simulink model "Progetto_PREDISTORTER_Aggiornato_15_021"  (R2024b)
settings: Solver=VariableStepAuto  StartTime=0.0  StopTime=10  RelTol=1e-3
libraries: commrflib2 x5, commfilt2 x1
settings Model: Creator=babu9  LastModifiedBy=Giorgio
settings SolverCC: AlgebraicLoopSolver=TrustRegion
settings RTWCC: GPUComputeCapability=3.5  DLArmComputeVersion=19.05

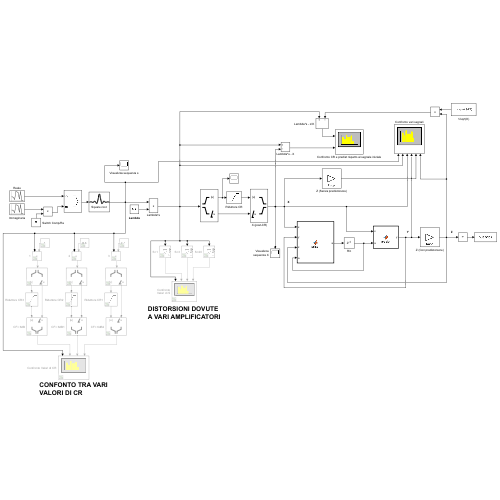
[thumbnail: Simulink's stored preview of the top-level diagram]
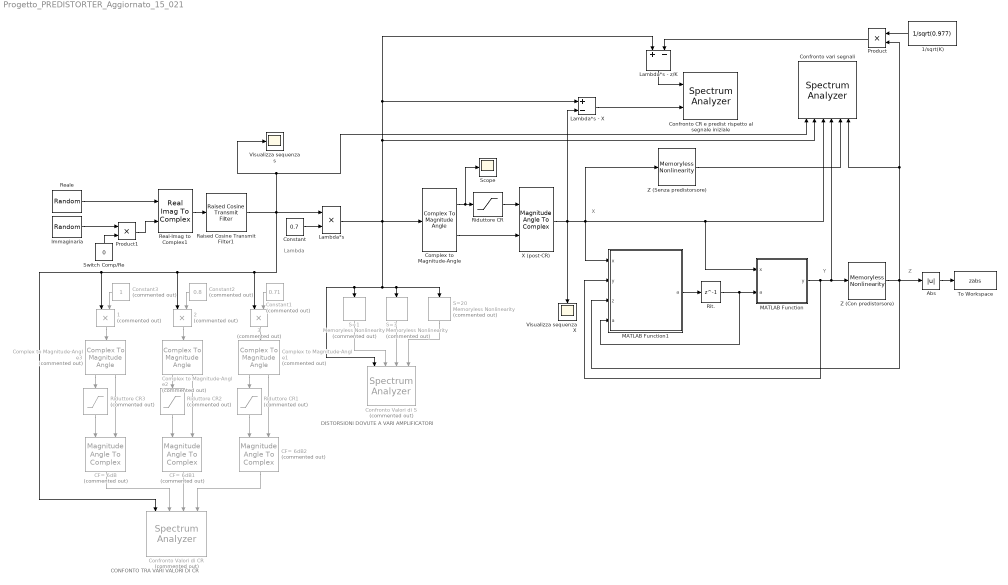
== system Progetto_PREDISTORTER_Aggiornato_15_021 ==
  note: DISTORSIONI DOVUTE
      | A VARI AMPLIFICATORI
  note: Lambda
  note: CONFONTO TRA VARI
      | VALORI DI CR
  note: Y
  note: Z
  note: X
  " X (post-CR)" : MagnitudeAngleToComplex
  1 : Product  Commented=on
  1/sqrt(K) : Constant  Value=1/sqrt(0.977)
  2 : Product  Commented=on
  3 : Product  Commented=on
  Abs : Abs  SaturateOnIntegerOverflow=off
  CF= 6dB : MagnitudeAngleToComplex  Commented=on
  CF= 6dB1 : MagnitudeAngleToComplex  Commented=on
  CF= 6dB2 : MagnitudeAngleToComplex  Commented=on
  Complex to Magnitude-Angle : ComplexToMagnitudeAngle
  Complex to Magnitude-Angle1 : ComplexToMagnitudeAngle  Commented=on
  Complex to Magnitude-Angle2 : ComplexToMagnitudeAngle  Commented=on
  Complex to Magnitude-Angle3 : ComplexToMagnitudeAngle  Commented=on
  Confronto Valori di S : SpectrumAnalyzer  Commented=on  NumInputPorts=4  AveragingMethod=Exponential  ShowLegend=on  ChannelNames="[\"\"]"  AllowFFTLengthLessThanSamplesPerUpdate=on  DefaultConfigurationName=spbscopes.SpectrumAnalyzerBlockCfg
  Confronto CR e predist rispetto al segnale iniziale : SpectrumAnalyzer  NumInputPorts=2  WindowPosition=[206.000000,154.000000,1536.000000,800.000000,]  ScopeFrameLocation=window  Span=8000  StartFrequency=-4000  StopFrequency=4000  AveragingMethod=Exponential  YLimits=[-58.97153624,-16.65787258]  ShowLegend=on  ChannelNames="[\"\"]"  AllowFFTLengthLessThanSamplesPerUpdate=on  DefaultConfigurationName=spbscopes.SpectrumAnalyzerBlockCfg
      settings: OpenAtSimulationStart=off
  Confronto Valori di CR : SpectrumAnalyzer  Commented=on  NumInputPorts=4  AveragingMethod=Exponential  ShowLegend=on  ChannelNames="[\"\"]"  AllowFFTLengthLessThanSamplesPerUpdate=on  DefaultConfigurationName=spbscopes.SpectrumAnalyzerBlockCfg
      settings: OpenAtSimulationStart=off
  Confronto vari segnali : SpectrumAnalyzer  NumInputPorts=6  WindowPosition=[257.000000,133.000000,1532.000000,791.000000,]  ScopeFrameLocation=window  SpectrumType=Power density  Span=80000  StartFrequency=-40000  StopFrequency=40000  AveragingMethod=Exponential  YLimits=[-146.14127615,3.33371478]  ShowLegend=on  ChannelNames="[\"s\", \"Lambda*s\", \"X post-CR\", \"Y (Uscita predistorsore)\", \"Z - Senza predistorsore\", \"Z - Con predistorsore\"]"  MeasurementChannel=3  AllowFFTLengthLessThanSamplesPerUpdate=on  DefaultConfigurationName=spbscopes.SpectrumAnalyzerBlockCfg
      settings: OpenAtSimulationStart=off
  Constant : Constant  Value=0.7
  Constant1 : Constant  Commented=on  Value=0.71
  Constant2 : Constant  Commented=on  Value=0.8
  Constant3 : Constant  Commented=on
  Immaginaria : RandomNumber  Seed=4387648932479  SampleTime=0.0001
  Lambda*s : Product
  Lambda*s - X : Sum  Inputs=+-
  Lambda*s - z/K : Sum  Inputs=+-
  MATLAB Function : MATLAB Function  TreatAsAtomicUnit=on
  MATLAB Function1 : MATLAB Function  TreatAsAtomicUnit=on
  Product : Product
  Product1 : Product
  Raised Cosine Transmit Filter1 : commfilt2/Raised Cosine Transmit Filter  filtType=Square root  R=0.25  filtSpan=100  N=8  filterGain=1  RateOptions=Allow multirate processing  framing=Mute  checkCoeff=off  variableName=TransmitFilter1  checkGain=Normalized  sampMode=Mute  saveAsFlag=0  currentFiltSpan=10  D=(10)/2  launchFVT=on  roundingMode=Floor  overflowMode=off  coeffDataTypeStr=Inherit: Same word length as input  coeffMin=[]  coeffMax=[]  coeffLastDataTypeStr=Inherit: Same word length as input  outputDataTypeStr=Inherit: Same as accumulator  outputMin=[]  outputMax=[]  outputLastDataTypeStr=Inherit: Same as accumulator
  Real-Imag to Complex1 : RealImagToComplex
  Reale : RandomNumber  Seed=3742346792324  SampleTime=0.0001
  Riduttore CR : Saturate  UpperLimit=1  LowerLimit=-1
  Riduttore CR1 : Saturate  Commented=on  UpperLimit=1  LowerLimit=-1
  Riduttore CR2 : Saturate  Commented=on  UpperLimit=1  LowerLimit=-1
  Riduttore CR3 : Saturate  Commented=on  UpperLimit=1  LowerLimit=-1
  Rit. : Delay  DelayLength=1  InitialCondition=ones(100,1)
  S=1 : commrflib2/Memoryless Nonlinearity  Commented=on  Model=modified-rapp  Gain=0  Nonlinearity=IIP3  IIP3=Inf  OIP3=Inf  IP1dB=Inf  OP1dB=Inf  IPsat=Inf  OPsat=Inf  Table=[ -25, 5, -1; -10, 20, -2; 0, 27, 5; 5, 28, 12 ]  MagnitudeGainDB=0  Vsat=1  MagnitudeSmooth=1  PhaseGainRadian=0  PhaseSaturation=1  PhaseSmooth=3.43  InputScaleDB=0  AmAmParameters=[ 2.1587, 1.1517 ]  AmPmParameters=[ 4.0033, 9.1040 ]  OutputScaleDB=0  ReferenceLoad=1  SimulateUsing=Code generation
  S=20 : commrflib2/Memoryless Nonlinearity  Commented=on  Model=modified-rapp  Gain=0  Nonlinearity=IIP3  IIP3=Inf  OIP3=Inf  IP1dB=Inf  OP1dB=Inf  IPsat=Inf  OPsat=Inf  Table=[ -25, 5, -1; -10, 20, -2; 0, 27, 5; 5, 28, 12 ]  MagnitudeGainDB=0  Vsat=1  MagnitudeSmooth=20  PhaseGainRadian=0  PhaseSaturation=1  PhaseSmooth=3.43  InputScaleDB=0  AmAmParameters=[ 2.1587, 1.1517 ]  AmPmParameters=[ 4.0033, 9.1040 ]  OutputScaleDB=0  ReferenceLoad=1  SimulateUsing=Code generation
  S=3 : commrflib2/Memoryless Nonlinearity  Commented=on  Model=modified-rapp  Gain=0  Nonlinearity=IIP3  IIP3=Inf  OIP3=Inf  IP1dB=Inf  OP1dB=Inf  IPsat=Inf  OPsat=Inf  Table=[ -25, 5, -1; -10, 20, -2; 0, 27, 5; 5, 28, 12 ]  MagnitudeGainDB=0  Vsat=1  MagnitudeSmooth=3  PhaseGainRadian=0  PhaseSaturation=1  PhaseSmooth=3.43  InputScaleDB=0  AmAmParameters=[ 2.1587, 1.1517 ]  AmPmParameters=[ 4.0033, 9.1040 ]  OutputScaleDB=0  ReferenceLoad=1  SimulateUsing=Code generation
  Scope : Scope
  Switch Comp/Re : Constant  Value=0
  To Workspace : ToWorkspace  VariableName=zabs  SampleTime=-1
      settings: Save2DSignal=2-D array (concatenate along first dimension)
  Visualizza sequenza X : Scope
  Visualizza sequenza s : Scope
  Z (Con predistorsore) : commrflib2/Memoryless Nonlinearity  Model=modified-rapp  Gain=0  Nonlinearity=IIP3  IIP3=Inf  OIP3=Inf  IP1dB=Inf  OP1dB=Inf  IPsat=Inf  OPsat=Inf  Table=[ -25, 5, -1; -10, 20, -2; 0, 27, 5; 5, 28, 12 ]  MagnitudeGainDB=0  Vsat=1  MagnitudeSmooth=3  PhaseGainRadian=0  PhaseSaturation=1  PhaseSmooth=3.43  InputScaleDB=0  AmAmParameters=[ 2.1587, 1.1517 ]  AmPmParameters=[ 4.0033, 9.1040 ]  OutputScaleDB=0  ReferenceLoad=1  SimulateUsing=Code generation
  Z (Senza predistorsore) : commrflib2/Memoryless Nonlinearity  Model=modified-rapp  Gain=0  Nonlinearity=IIP3  IIP3=Inf  OIP3=Inf  IP1dB=Inf  OP1dB=Inf  IPsat=Inf  OPsat=Inf  Table=[ -25, 5, -1; -10, 20, -2; 0, 27, 5; 5, 28, 12 ]  MagnitudeGainDB=0  Vsat=1  MagnitudeSmooth=3  PhaseGainRadian=0  PhaseSaturation=1  PhaseSmooth=3.43  InputScaleDB=0  AmAmParameters=[ 2.1587, 1.1517 ]  AmPmParameters=[ 4.0033, 9.1040 ]  OutputScaleDB=0  ReferenceLoad=1  SimulateUsing=Code generation
  wires:
  Reale/1 -> Real-Imag to Complex1/1
  Riduttore CR/1 -> " X (post-CR)"/1
  Complex to Magnitude-Angle/1 -> Scope/1, Riduttore CR/1
  Complex to Magnitude-Angle/2 -> " X (post-CR)"/2
  Z (Con predistorsore)/1 -> Confronto vari segnali/6, Product/2, Abs/1, MATLAB Function1/3(z)
  Immaginaria/1 -> Product1/1
  Switch Comp/Re/1 -> Product1/2
  Product1/1 -> Real-Imag to Complex1/2
  S=1/1 -> Confronto Valori di S/2
  S=3/1 -> Confronto Valori di S/3
  S=20/1 -> Confronto Valori di S/4
  Abs/1 -> To Workspace/1
  Lambda*s/1 -> Confronto vari segnali/2, Lambda*s - X/1, Lambda*s - z/K/1, Complex to Magnitude-Angle/1, Confronto Valori di S/1, S=1/1, S=20/1, S=3/1
  1/sqrt(K)/1 -> Product/1
  Product/1 -> Lambda*s - z/K/2
  Lambda*s - z/K/1 -> Confronto CR e predist rispetto al segnale iniziale/1
  Lambda*s - X/1 -> Confronto CR e predist rispetto al segnale iniziale/2
  Complex to Magnitude-Angle1/2 -> CF= 6dB2/2
  CF= 6dB1/1 -> Confronto Valori di CR/3
  Complex to Magnitude-Angle2/2 -> CF= 6dB1/2
  3/1 -> Complex to Magnitude-Angle1/1
  CF= 6dB2/1 -> Confronto Valori di CR/4
  CF= 6dB/1 -> Confronto Valori di CR/2
  Riduttore CR1/1 -> CF= 6dB2/1
  Complex to Magnitude-Angle3/2 -> CF= 6dB/2
  Riduttore CR2/1 -> CF= 6dB1/1
  Complex to Magnitude-Angle3/1 -> Riduttore CR3/1
  Complex to Magnitude-Angle1/1 -> Riduttore CR1/1
  Complex to Magnitude-Angle2/1 -> Riduttore CR2/1
  Constant1/1 -> 3/2
  1/1 -> Complex to Magnitude-Angle3/1
  2/1 -> Complex to Magnitude-Angle2/1
  Riduttore CR3/1 -> CF= 6dB/1
  Constant3/1 -> 1/2
  Constant2/1 -> 2/2
  Raised Cosine Transmit Filter1/1 -> Visualizza sequenza s/1, Confronto vari segnali/1, Lambda*s/1, 2/1, 1/1, Confronto Valori di CR/1, 3/1
  Real-Imag to Complex1/1 -> Raised Cosine Transmit Filter1/1
  " X (post-CR)"/1 -> Lambda*s - X/2, Z (Senza predistorsore)/1, Confronto vari segnali/3, MATLAB Function/1(x), MATLAB Function1/1(x), Visualizza sequenza X/1
  Z (Senza predistorsore)/1 -> Confronto vari segnali/5
  MATLAB Function1/1(a) -> Rit./1
  MATLAB Function/1(y) -> Z (Con predistorsore)/1, Confronto vari segnali/4, MATLAB Function1/2(y)
  Rit./1 -> MATLAB Function/2(a), MATLAB Function1/4("a ")
  Constant/1 -> Lambda*s/2

== matlab function Progetto_PREDISTORTER_Aggiornato_15_021/MATLAB Function1 ==
  data: x input; a output; y input; z input; a input
function a = adapt(x,y,z,a)

N=64;                         % Number of intervals
gamma=0.005;                  % Step size
xmax=1;                       % Max scale value
K=sqrt(0.977);                % Predistortion gain
delta=xmax/N;                 % Intervals amplitude
int_vec=0:delta:xmax;         % Interval vector
n=zeros(1,length(int_vec));   % Positioning vector for every sample of the sequence aprec (size N+1)

if abs(x)>=xmax
   n(end)=1;
end
aux=find(abs(x)>int_vec);     % n contains 1 for x>int_vec(n) 
n(aux(end))=1;                % Last index is the last value below x: it's the interval!

index_vec=find(n);
index=index_vec(1);

a(index)=real(a(index) - gamma * (z-K*x) * conj(x*z/y)); % From theory

end

% If |x|>xmax, the value x is mapped as the last of the N+1 ordinates a for adaption.
% Otherwise, an auxiliary variable aux is used in order to store the indices i of int_vec for which the condition |x|>int_vec(i) 
% is satisfied. Between all the obtained indices, the last one is taken as it corresponds to the index of the correct interval to
% be used for the mapping (from x to a).

% WARNING: do not encrease N over 99 without changing the initial conditions of Rit.

== matlab function Progetto_PREDISTORTER_Aggiornato_15_021/MATLAB Function ==
  data: x input; a input; y output
function y = predist(x,a)

N = 64;                         % Number of intervals
xmax = 1;                       % Max scale value
delta = xmax/N;                 % Intervals amplitude
int_vec = 0:delta:xmax;         % Interval vector
n = zeros(1,length(int_vec));   % Positioning vector for every sample of the sequence a

if (abs(x)>xmax)
    n(end)=1;                   % Saturation: x>xmax
end
aux=find(abs(x)>int_vec);       % n contains 1 for x>int_vec(n)
n(aux(end))=1;                  % Last index is the last value below x: it's the interval!

index_vec=find(n);
index=index_vec(1);

P=1/(2*delta)*((abs(x)-(2*index+1)*delta)*(a(index+1)-a(index))) + 1/2*(a(index+1)+a(index));

y=P*x;

end

% If |x|>xmax, the value x is mapped as the last of the N+1 ordinates a for adaption.
% Otherwise, an auxiliary variable aux is used in order to store the indices i of int_vec for which the condition |x|>int_vec(i) 
% is satisfied. Between all the obtained indices, the last one is taken as it corresponds to the index of the correct interval to
% be used for the mapping (from x to a).

% WARNING: do not encrease N over 99 without changing the initial conditions of Rit.

% Predistortion is obtained via piece-wise linear interpolation between the N+1 ordinates a generated from the mapping described
% in the code for block "adapt".
